simulink model "Ros2_link"  (R2024a)
settings: Solver=FixedStepAuto  StartTime=0.0  StopTime=inf  RelTol=1e-3
libraries: ros2lib x3
settings Model: Creator=The MathWorks, Inc.  LastModifiedBy=farall
settings SolverCC: AlgebraicLoopSolver=TrustRegion
settings OptimizationCC: EnhancedBackFolding=on  PassReuseOutputArgsAs=Individual arguments  ZeroExternalMemoryAtStartup=off  ZeroInternalMemoryAtStartup=off  MaxStackSize=64  OptimizeBlockOrder=speed  DifferentSizesBufferReuse=on  OptimizationCustomize=off  EfficientTunableParamExpr=on
settings DebuggingCC: ParameterTunabilityLossMsg=error  UnconnectedInputMsg=warning  UnconnectedOutputMsg=warning  UnconnectedLineMsg=warning  SymbolicDimsDataTypeCodeGenerationDiagnostic=none
settings ModelReferenceCC: EnableRefExpFcnMdlSchedulingChecks=on
settings SFSimCC: MATLABDynamicMemAlloc=off  SimTargetLang=C++
settings RTWCC: Description=Embedded Coder  SystemTargetFile=ert.tlc  HardwareBoard=Robot Operating System 2 (ROS 2)  TemplateMakefile=ert_default_tmf  GenerateReport=on  Toolchain=Colcon Tools  IncludeHyperlinkInReport=on  LaunchReport=on  TargetLang=C++  GenerateTraceInfo=on  GenerateTraceReport=on  GenerateTraceReportSl=on  GenerateTraceReportSf=on  GenerateTraceReportEml=on  GPUComputeCapability=3.5
settings CodeAppCC: ForceParamTrailComments=on  IgnoreCustomStorageClasses=off  OperatorAnnotations=on  SimulinkDataObjDesc=on  SFDataObjDesc=on  InsertBlockDesc=on
settings ERTTargetCC: CodeInterfacePackaging=C++ class  RootIOFormat=Structure reference

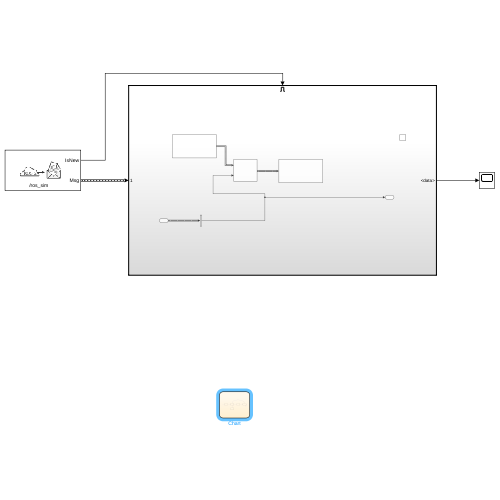
[thumbnail: Simulink's stored preview of the top-level diagram]
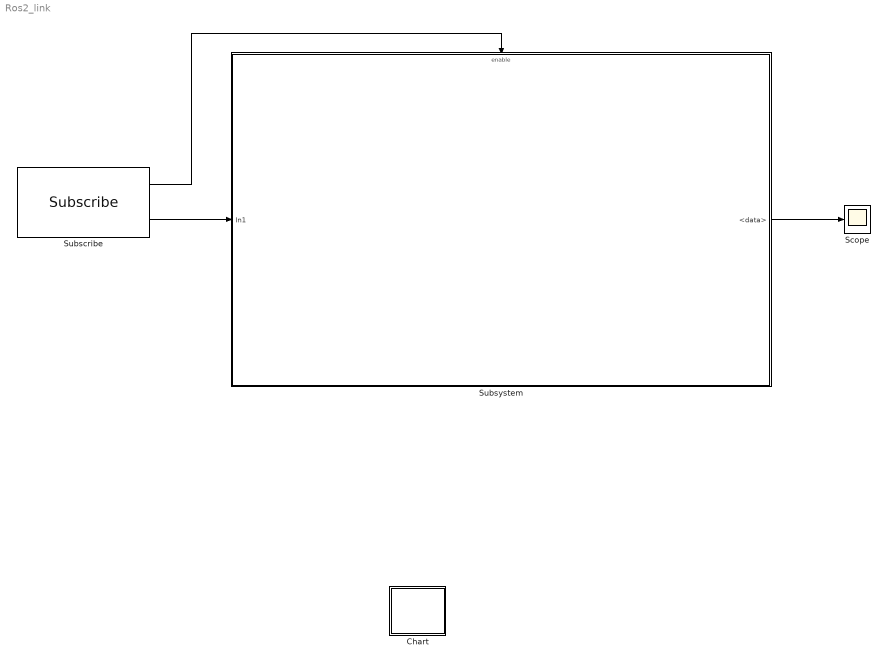
== system Ros2_link ==
  Chart : Stateflow chart  TreatAsAtomicUnit=on
  Scope : Scope
  Subscribe : ros2lib/Subscribe  topicSource=Specify your own  topic=/ros_sim  messageType=std_msgs/UInt8  sampleTime=-1  QOSHistory=Keep last  QOSDepth=1  QOSReliability=Reliable  QOSDurability=Volatile  QOSDeadline=Inf  QOSLifespan=Inf  QOSLiveliness=Automatic  QOSLeaseDuration=Inf  QOSAvoidROSNamespaceConventions=off
  Subsystem : Subsystem
  wires:
  Subscribe/1 -> Subsystem/Enable
  Subscribe/2 -> Subsystem/1(In1)
  Subsystem/1(<data>) -> Scope/1

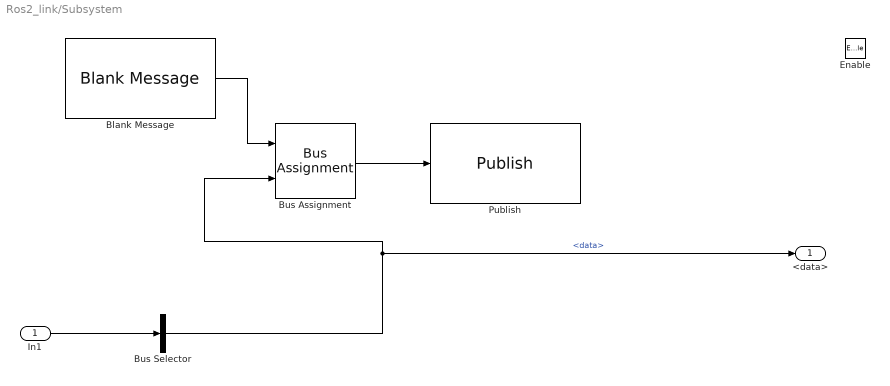
== system Ros2_link/Subsystem ==
  In1 : Inport
  Enable : EnablePort
  Blank Message : ros2lib/Blank Message  messageClass=Message  entityType=std_msgs/UInt8  messageType=std_msgs/UInt8  SampleTime=0.01
  Bus Assignment : BusAssignment  AssignedSignals=data
  Bus Selector : BusSelector  OutputSignals=data
  Publish : ros2lib/Publish  topicSource=Specify your own  topic=/sim_ros  messageType=std_msgs/UInt8  QOSHistory=Keep last  QOSDepth=1  QOSReliability=Reliable  QOSDurability=Volatile  QOSDeadline=Inf  QOSLifespan=Inf  QOSLiveliness=Automatic  QOSLeaseDuration=Inf  QOSAvoidROSNamespaceConventions=off
  <data> : Outport
  wires:
  Blank Message/1 -> Bus Assignment/1
  Bus Assignment/1 -> Publish/1
  Bus Selector/1 -> <data>/1, Bus Assignment/2  "<data>"
  In1/1 -> Bus Selector/1

== stateflow chart Ros2_link/Chart ==
  state Init
  state Home
  state Approach
  state Stroke
  state End
  state Error
  Stroke -> Home [order 2]
  Init -> Home [order 1]
  Home -> Approach [order 1]
  Approach -> Stroke [order 1]
  (default) -> Init
  Stroke -> Stroke [order 1]
  Init -> Error [order 2]
  Home -> End [order 2]
  Approach -> Error [order 2]
